simulink model "hcu_main_ADASwEPS"  (Simulink 8.2)
settings: Solver=FixedStepDiscrete  StartTime=0.0  StopTime=inf  FixedStep=0.001  RelTol=1e-3
PostLoadFcn:
  | , if any(exist('dsrtsu_mdlpostloadfcn', 'file') == [2, 3, 6]), try dsrtsu_mdlpostloadfcn('Execute', bdroot); catch fprintf('Error in PostLoadFcn (dsrtsu_mdlpostloadfcn) for model "%s":\n %s\n', bdroot, lasterr); end, end,
values from neighbouring files (symbols this model uses):
  C_TASK_1MS_S = (	C_TICK_TIME_S       )    [hcu_local_hdr.m]    (also in temp_ovrd_values.m = double(	0.001                  ))
  C_TICK_TIME_S = single(	0.005	    	)    [hcu_local_hdr.m]
  ENUM_EPSLFCSTATUS_ACTIVE = uint8(  2  )    [hcu_local_hdr.m]
  ENUM_EPSLFCSTATUS_TRANSITION = uint8(  3  )    [hcu_local_hdr.m]
  ENUM_EPSLKASTATUS_ACTIVE = uint8(  2  )    [hcu_local_hdr.m]
  ENUM_EPSMODEREQ_ANGLE = uint8(  1  )    [hcu_local_hdr.m]
  ENUM_EPSMODEREQ_INTERNAL = uint8(  0  )    [hcu_local_hdr.m]
  ENUM_EPSMODEREQ_TORQUE = uint8(  2  )    [hcu_local_hdr.m]
  ENUM_GEARPOSN_1ST = uint8(  1  )    [hcu_local_hdr.m]
  ENUM_GEARPOSN_2ND = uint8(  2  )    [hcu_local_hdr.m]
  ENUM_GEARPOSN_3RD = uint8(  3  )    [hcu_local_hdr.m]
  ENUM_GEARPOSN_4TH = uint8(  4  )    [hcu_local_hdr.m]
  ENUM_GEARPOSN_5TH = uint8(  5  )    [hcu_local_hdr.m]
  ENUM_GEARPOSN_6TH = uint8(  6  )    [hcu_local_hdr.m]
  ENUM_GEARPOSN_R = uint8(  7  )    [hcu_local_hdr.m]
  FALSE = boolean( 0 )    [hcu_local_hdr.m]
  TRUE = boolean( 1 )    [hcu_local_hdr.m]
undefined symbols (not defined in the file or in its folder): AISP_EPSCurrent_pct, AISP_TqASensorDelta_pct, AISP_TqBSensorDelta_pct, dHAL_IN, hal, INVALID_ABS1_TIMEOUT, INVALID_ABS2_TIMEOUT, INVALID_ABS3_TIMEOUT, INVALID_ABS4_TIMEOUT, INVALID_AC1_TIMEOUT, INVALID_ADASTORQ_REQ, INVALID_BCM1_TIMEOUT, INVALID_BCM2_TIMEOUT, INVALID_BOOSTER_VAC, INVALID_CSW1_TIMEOUT, INVALID_CUR_VEHDECE, INVALID_CURBRAKEDECE_REQ, INVALID_CURSTEERANG_REQ, INVALID_CURSTEERTQ_REQ, INVALID_ECM1_TIMEOUT, INVALID_ECM2_TIMEOUT, INVALID_ECM3_TIMEOUT, INVALID_ECM9_TIMEOUT, INVALID_ENG_TORQUE_FRICTIONAL, INVALID_ENG_TORQUE_INDICATED, INVALID_ENG_TORQUE_INDICATEDCOR, INVALID_ENG_TQ_MAX, INVALID_ENG_TQ_MIN, INVALID_EPAS2_TIMEOUT, INVALID_EPAS3_TIMEOUT, INVALID_EPB1_TIMEOUT, INVALID_EPS_BATTVOLT, INVALID_ESC_BATTVOLT, INVALID_GRADE, INVALID_HCU3_TIMEOUT, INVALID_HCU4_TIMEOUT, INVALID_HMI1_TIMEOUT, INVALID_HMI2_TIMEOUT, INVALID_LAT_ACC, INVALID_LONG_ACC, INVALID_MC_PRESSURE, INVALID_METER1_TIMEOUT, INVALID_METER3_TIMEOUT, INVALID_METER_VEHSPD, INVALID_ODO_METER, INVALID_OUTSIDE_TEMP, INVALID_PARKBRAKEBIND_STAT, INVALID_PEDALTQ_REQ, INVALID_SAS1_TIMEOUT, INVALID_SAS_ANGLE, INVALID_SHIFTER_POSN, INVALID_TCM1_TIMEOUT, INVALID_TCM2_TIMEOUT, INVALID_VCU1_TIMEOUT, INVALID_VCU2_TIMEOUT, INVALID_VEH_CRASH, INVALID_VEH_SPD, INVALID_WHEEL_SPD, INVALID_YAW_RATE, KHAL_MssgIdObj1_num ... (+8)
libraries: simulink x147, hcu_lib x38, rti1401lib_dio_type3 x4, rtimmsu_dsrtlib x3, app x1, rtiethernetudplib x1, rti1401lib_adc_type4 x1, rti1401lib_dac_type3 x1, inp x1, lidr x1, outp x1
(part 15 of 15)

== stateflow chart EPSS/EPSS/InternalMode/LKA_Flow_Chart ==
  state UNAVAILABLE
    VEPSS_EPSLKAStatus_enum=ENUM_EPSLKASTATUS_OFF;
  state AVAILABLE
    VEPSS_EPSLKAStatus_enum=ENUM_EPSLKASTATUS_READY;
  state PROGRESS
    VEPSS_EPSLKAStatus_enum=ENUM_EPSLKASTATUS_ACTIVE;
  state INVALID
    VEPSS_EPSLKAStatus_enum=ENUM_EPSLKASTATUS_NOTAVAIL_PERM;
  (default) -> UNAVAILABLE : {VEPSS_EPSLKAAbReason_enum= ...
      | ENUM_EPSADASABREASON_NO_DRIVING_INTERRUPTION;}
  AVAILABLE -> PROGRESS [order 2] : [VISP_ADASLKAStatus_enum==ENUM_ADASLKASTATUS_ACTIVE && ...
      | VISP_EPSModeReq_enum==ENUM_EPSMODEREQ_INTERNAL && ...
      | VISP_StrTqReqAppl_flg]
      | {VEPSS_EPSLKAAbReason_enum= ...
      | ENUM_EPSADASABREASON_NO_DRIVING_INTERRUPTION;}
  UNAVAILABLE -> AVAILABLE [order 1] : [VISP_ADASLKAStatus_enum==ENUM_ADASLKASTATUS_STANDBY && ...
      | VISP_EPSModeReq_enum==ENUM_EPSMODEREQ_INTERNAL]
      | {VEPSS_EPSLKAAbReason_enum= ...
      | ENUM_EPSADASABREASON_NO_DRIVING_INTERRUPTION;}
  PROGRESS -> AVAILABLE [order 1] : [VISP_EPSModeReq_enum==ENUM_EPSMODEREQ_INTERNAL && ...
      | (VISP_ADASLKAStatus_enum==ENUM_ADASLKASTATUS_STANDBY || ...
      | !VISP_StrTqReqAppl_flg)]
      | {VEPSS_EPSLKAAbReason_enum= ...
      | ENUM_EPSADASABREASON_NO_DRIVING_INTERRUPTION;}
  AVAILABLE -> UNAVAILABLE [order 1] : [(VISP_ADASLKAStatus_enum==ENUM_ADASLKASTATUS_OFF || ...
      | VISP_EPSModeReq_enum==ENUM_EPSMODEREQ_TORQUE || ...
      | VISP_EPSModeReq_enum==ENUM_EPSMODEREQ_ANGLE)]
      | {VEPSS_EPSLKAAbReason_enum= ...
      | ENUM_EPSADASABREASON_NO_DRIVING_INTERRUPTION;}
  (junction 314) -> UNAVAILABLE
  (junction 313) -> UNAVAILABLE
  UNAVAILABLE -> (junction 311) [order 2]
  AVAILABLE -> INVALID [order 3] : [VISP_ADASLKAStatus_enum==ENUM_ADASLKASTATUS_NOTAVAIL_TEMP || ...
      | VISP_ADASLKAStatus_enum==ENUM_ADASLKASTATUS_NOTAVAIL_PERM || ...
      | VISP_EPSModeReq_enum==ENUM_EPSMODEREQ_INVALID]
      | {VEPSS_EPSLKAAbReason_enum= ...
      | ENUM_EPSADASABREASON_OTHER_DEFAULT;}
  PROGRESS -> (junction 312) [order 2]
  PROGRESS -> (junction 315) [order 3]
  (junction 311) -> INVALID : [VISP_ADASLKAStatus_enum==ENUM_ADASLKASTATUS_NOTAVAIL_TEMP || ...
      | VISP_ADASLKAStatus_enum==ENUM_ADASLKASTATUS_NOTAVAIL_PERM || ...
      | VISP_EPSModeReq_enum==ENUM_EPSMODEREQ_INVALID]
      | {VEPSS_EPSLKAAbReason_enum= ...
      | ENUM_EPSADASABREASON_OTHER_DEFAULT;}
  (junction 312) -> INVALID : [VISP_ADASLKAStatus_enum==ENUM_ADASLKASTATUS_NOTAVAIL_TEMP || ...
      | VISP_ADASLKAStatus_enum==ENUM_ADASLKASTATUS_NOTAVAIL_PERM || ...
      | VISP_EPSModeReq_enum==ENUM_EPSMODEREQ_INVALID]
      | {VEPSS_EPSLKAAbReason_enum= ...
      | ENUM_EPSADASABREASON_OTHER_DEFAULT;}
  INVALID -> (junction 313) : [VISP_ADASLKAStatus_enum==ENUM_ADASLKASTATUS_OFF && ...
      | VEPSS_StrTqReqZERO_flg]
      | {VEPSS_EPSLKAAbReason_enum= ...
      | ENUM_EPSADASABREASON_NO_DRIVING_INTERRUPTION;}
  (junction 315) -> (junction 314) : [(VISP_ADASLKAStatus_enum==ENUM_ADASLKASTATUS_OFF || ...
      | VISP_EPSModeReq_enum==ENUM_EPSMODEREQ_TORQUE || ...
      | VISP_EPSModeReq_enum==ENUM_EPSMODEREQ_ANGLE)]
      | {VEPSS_EPSLKAAbReason_enum= ...
      | ENUM_EPSADASABREASON_NO_DRIVING_INTERRUPTION;}
  data: VEPSS_EPSLKAStatus_enum output uint8; ENUM_EPSLKASTATUS_OFF parameter double; ENUM_EPSLKASTATUS_READY parameter double; ENUM_EPSLKASTATUS_ACTIVE parameter double; ENUM_EPSLKASTATUS_NOTAVAIL_TEMP parameter double; ENUM_EPSLKASTATUS_NOTAVAIL_PERM parameter double; VISP_ADASLKAStatus_enum input double; ENUM_ADASLKASTATUS_OFF parameter double; ENUM_ADASLKASTATUS_STANDBY parameter double; ENUM_ADASLKASTATUS_ACTIVE parameter double; ENUM_ADASLKASTATUS_NOTAVAIL_TEMP parameter double; ENUM_ADASLKASTATUS_NOTAVAIL_PERM parameter double; VISP_EPSModeReq_enum input double; VEPSS_StrTqReqZERO_flg input double; ENUM_EPSMODEREQ_INTERNAL parameter double; ENUM_EPSMODEREQ_ANGLE parameter double; ENUM_EPSMODEREQ_TORQUE parameter double; ENUM_EPSMODEREQ_INVALID parameter double; VEPSS_EPSLKAAbReason_enum output uint8; ENUM_EPSADASABREASON_NO_DRIVING_INTERRUPTION parameter double; ENUM_EPSADASABREASON_THERMAL_ERROR parameter double; ENUM_EPSADASABREASON_GEAR_POSITION_ERROR parameter double; ENUM_EPSADASABREASON_VEHICLE_SPEED_ERROR parameter double; ENUM_EPSADASABREASON_DRIVER_RECOVERY parameter double; ENUM_EPSADASABREASON_TORQUE_ERROR parameter double; ENUM_EPSADASABREASON_REQUEST_TORQUE_ERROR parameter double; ENUM_EPSADASABREASON_THERMAL_PROTECTION parameter double; ENUM_EPSADASABREASON_TRANSITION_GAIN_ERROR parameter double; ENUM_EPSADASABREASON_OTHER_DEFAULT parameter double; VISP_StrTqReqAppl_flg input double

== stateflow chart EPSS/EPSS/TorqueMode/LFC_Flow_Chart ==
  state UNAVAILABLE
    VEPSS_EPSLFCStatus_enum=ENUM_EPSLFCSTATUS_OFF;
  state AVAILABLE
    VEPSS_EPSLFCStatus_enum=ENUM_EPSLFCSTATUS_READY;
  state PROGRESS_NORMAL
    VEPSS_EPSLFCStatus_enum=ENUM_EPSLFCSTATUS_ACTIVE;
  state INVALID
    VEPSS_EPSLFCStatus_enum=ENUM_EPSLFCSTATUS_NOTAVAIL_PERM;
  state PROGRESS_TRANSITION
    VEPSS_EPSLFCStatus_enum=ENUM_EPSLFCSTATUS_TRANSITION;
  (default) -> UNAVAILABLE : {VEPSS_EPSLFCAbReason_enum= ...
      | ENUM_EPSADASABREASON_NO_DRIVING_INTERRUPTION;}
  AVAILABLE -> PROGRESS_NORMAL [order 2] : [VISP_ADASLFCStatus_enum==ENUM_ADASLFCSTATUS_ACTIVE_NORMAL && ...
      | VISP_EPSModeReq_enum==ENUM_EPSMODEREQ_TORQUE && ...
      | VISP_StrTqReqAppl_flg]
      | {VEPSS_EPSLFCAbReason_enum= ...
      | ENUM_EPSADASABREASON_NO_DRIVING_INTERRUPTION;}
  UNAVAILABLE -> AVAILABLE [order 1] : [VISP_ADASLFCStatus_enum==ENUM_ADASLFCSTATUS_STANDBY]
      | {VEPSS_EPSLFCAbReason_enum= ...
      | ENUM_EPSADASABREASON_NO_DRIVING_INTERRUPTION;}
  PROGRESS_NORMAL -> (junction 371) [order 4] : [VISP_ADASLFCStatus_enum==ENUM_ADASLFCSTATUS_OFF]
      | {VEPSS_EPSLFCAbReason_enum= ...
      | ENUM_EPSADASABREASON_NO_DRIVING_INTERRUPTION;}
  (junction 371) -> (junction 386)
  PROGRESS_NORMAL -> AVAILABLE [order 1] : [(VISP_ADASLFCStatus_enum==ENUM_ADASLFCSTATUS_STANDBY || ...
      | VISP_EPSModeReq_enum==ENUM_EPSMODEREQ_INTERNAL || ...
      | VISP_EPSModeReq_enum==ENUM_EPSMODEREQ_ANGLE || ...
      | !VISP_StrTqReqAppl_flg)]
      | {VEPSS_EPSLFCAbReason_enum= ...
      | ENUM_EPSADASABREASON_NO_DRIVING_INTERRUPTION;}
  AVAILABLE -> UNAVAILABLE [order 1] : [VISP_ADASLFCStatus_enum==ENUM_ADASLFCSTATUS_OFF]
      | {VEPSS_EPSLFCAbReason_enum= ...
      | ENUM_EPSADASABREASON_NO_DRIVING_INTERRUPTION;}
  (junction 384) -> UNAVAILABLE
  (junction 382) -> UNAVAILABLE
  UNAVAILABLE -> (junction 378) [order 2]
  AVAILABLE -> (junction 374) [order 3]
  (junction 372) -> AVAILABLE
  PROGRESS_NORMAL -> (junction 379) [order 2]
  PROGRESS_NORMAL -> PROGRESS_TRANSITION [order 3] : [VISP_ADASLFCStatus_enum==ENUM_ADASLFCSTATUS_ACTIVE_TRANSITION && ...
      | VISP_EPSModeReq_enum==ENUM_EPSMODEREQ_TORQUE && ...
      | VISP_StrTqReqAppl_flg]
      | {VEPSS_EPSLFCAbReason_enum= ...
      | ENUM_EPSADASABREASON_NO_DRIVING_INTERRUPTION;}
  PROGRESS_TRANSITION -> (junction 372) [order 3] : [(VISP_ADASLFCStatus_enum==ENUM_ADASLFCSTATUS_STANDBY || ...
      | VISP_EPSModeReq_enum==ENUM_EPSMODEREQ_INTERNAL || ...
      | VISP_EPSModeReq_enum==ENUM_EPSMODEREQ_ANGLE || ...
      | !VISP_StrTqReqAppl_flg)]
      | {VEPSS_EPSLFCAbReason_enum= ...
      | ENUM_EPSADASABREASON_NO_DRIVING_INTERRUPTION;}
  PROGRESS_TRANSITION -> (junction 373) [order 1] : [VISP_ADASLFCStatus_enum==ENUM_ADASLFCSTATUS_OFF]
      | {VEPSS_EPSLFCAbReason_enum= ...
      | ENUM_EPSADASABREASON_NO_DRIVING_INTERRUPTION;}
  (junction 373) -> (junction 385)
  (junction 374) -> (junction 375) [order 1] : [!VEPSS_LFCTransGainONE_flg]
      | {VEPSS_EPSLFCAbReason_enum= ...
      | ENUM_EPSADASABREASON_TRANSITION_GAIN_ERROR;}
  (junction 374) -> (junction 376) [order 2]
  (junction 375) -> (junction 377)
  PROGRESS_TRANSITION -> (junction 383) [order 2]
  (junction 376) -> (junction 377) : [VISP_ADASLFCStatus_enum==ENUM_ADASLFCSTATUS_NOTAVAIL_TEMP || ...
      | VISP_ADASLFCStatus_enum==ENUM_ADASLFCSTATUS_NOTAVAIL_PERM || ...
      | VISP_EPSModeReq_enum==ENUM_EPSMODEREQ_INVALID]
      | {VEPSS_EPSLFCAbReason_enum= ...
      | ENUM_EPSADASABREASON_OTHER_DEFAULT;}
  (junction 377) -> INVALID
  (junction 378) -> INVALID [order 1] : [!VEPSS_LFCTransGainONE_flg]
      | {VEPSS_EPSLFCAbReason_enum= ...
      | ENUM_EPSADASABREASON_TRANSITION_GAIN_ERROR;}
  (junction 379) -> INVALID [order 1] : [!VEPSS_LFCTransGainONE_flg]
      | {VEPSS_EPSLFCAbReason_enum= ...
      | ENUM_EPSADASABREASON_TRANSITION_GAIN_ERROR;}
  (junction 378) -> (junction 380) [order 2]
  (junction 379) -> (junction 381) [order 2]
  (junction 380) -> INVALID : [VISP_ADASLFCStatus_enum==ENUM_ADASLFCSTATUS_NOTAVAIL_TEMP || ...
      | VISP_ADASLFCStatus_enum==ENUM_ADASLFCSTATUS_NOTAVAIL_PERM || ...
      | VISP_EPSModeReq_enum==ENUM_EPSMODEREQ_INVALID]
      | {VEPSS_EPSLFCAbReason_enum= ...
      | ENUM_EPSADASABREASON_OTHER_DEFAULT;}
  (junction 381) -> INVALID : [VISP_ADASLFCStatus_enum==ENUM_ADASLFCSTATUS_NOTAVAIL_TEMP || ...
      | VISP_ADASLFCStatus_enum==ENUM_ADASLFCSTATUS_NOTAVAIL_PERM || ...
      | VISP_EPSModeReq_enum==ENUM_EPSMODEREQ_INVALID]
      | {VEPSS_EPSLFCAbReason_enum= ...
      | ENUM_EPSADASABREASON_OTHER_DEFAULT;}
  INVALID -> (junction 382) : [VISP_ADASLFCStatus_enum==ENUM_ADASLFCSTATUS_OFF && ...
      | VEPSS_StrTqReqZERO_flg && ...
      | VEPSS_LFCTransGainONE_flg]
      | {VEPSS_EPSLFCAbReason_enum= ...
      | ENUM_EPSADASABREASON_NO_DRIVING_INTERRUPTION;}
  (junction 383) -> INVALID : [VISP_ADASLFCStatus_enum==ENUM_ADASLFCSTATUS_NOTAVAIL_TEMP || ...
      | VISP_ADASLFCStatus_enum==ENUM_ADASLFCSTATUS_NOTAVAIL_PERM || ...
      | VISP_EPSModeReq_enum==ENUM_EPSMODEREQ_INVALID]
      | {VEPSS_EPSLFCAbReason_enum= ...
      | ENUM_EPSADASABREASON_OTHER_DEFAULT;}
  (junction 385) -> (junction 384)
  (junction 386) -> (junction 385)
  data: VEPSS_EPSLFCStatus_enum output uint8; ENUM_EPSLFCSTATUS_OFF parameter double; ENUM_EPSLFCSTATUS_READY parameter double; ENUM_EPSLFCSTATUS_ACTIVE parameter double; ENUM_EPSLFCSTATUS_NOTAVAIL_TEMP parameter double; ENUM_EPSLFCSTATUS_NOTAVAIL_PERM parameter double; VISP_ADASLFCStatus_enum input double; ENUM_ADASLFCSTATUS_OFF parameter double; ENUM_ADASLFCSTATUS_STANDBY parameter double; ENUM_ADASLFCSTATUS_ACTIVE_NORMAL parameter double; ENUM_ADASLFCSTATUS_NOTAVAIL_TEMP parameter double; ENUM_ADASLFCSTATUS_NOTAVAIL_PERM parameter double; VISP_EPSModeReq_enum input double; VISP_StrTqReqAppl_flg input double; VEPSS_StrTqReqZERO_flg input double; ENUM_EPSMODEREQ_INTERNAL parameter double; ENUM_EPSMODEREQ_ANGLE parameter double; ENUM_EPSMODEREQ_TORQUE parameter double; ENUM_EPSMODEREQ_INVALID parameter double; VEPSS_EPSLFCAbReason_enum output uint8; ENUM_EPSADASABREASON_NO_DRIVING_INTERRUPTION parameter double; ENUM_EPSADASABREASON_THERMAL_ERROR parameter double; ENUM_EPSADASABREASON_GEAR_POSITION_ERROR parameter double; ENUM_EPSADASABREASON_VEHICLE_SPEED_ERROR parameter double; ENUM_EPSADASABREASON_DRIVER_RECOVERY parameter double; ENUM_EPSADASABREASON_TORQUE_ERROR parameter double; ENUM_EPSADASABREASON_REQUEST_TORQUE_ERROR parameter double; ENUM_EPSADASABREASON_THERMAL_PROTECTION parameter double; ENUM_EPSADASABREASON_TRANSITION_GAIN_ERROR parameter double; ENUM_EPSADASABREASON_OTHER_DEFAULT parameter double; ENUM_EPSLFCSTATUS_TRANSITION parameter double; ENUM_ADASLFCSTATUS_ACTIVE_TRANSITION parameter double; VEPSS_LFCTransGainONE_flg input double

== stateflow chart EPSS/EPSS/AngleMode/LFC_Flow_Chart ==
  state UNAVAILABLE
    VEPSS_EPSLFCStatus_enum=ENUM_EPSLFCSTATUS_OFF;
  state AVAILABLE
    VEPSS_EPSLFCStatus_enum=ENUM_EPSLFCSTATUS_READY;
  state PROGRESS_NORMAL
    VEPSS_EPSLFCStatus_enum=ENUM_EPSLFCSTATUS_ACTIVE;
  state INVALID
    VEPSS_EPSLFCStatus_enum=ENUM_EPSLFCSTATUS_NOTAVAIL_PERM;
  state PROGRESS_TRANSITION
    VEPSS_EPSLFCStatus_enum=ENUM_EPSLFCSTATUS_TRANSITION;
  (default) -> UNAVAILABLE : {VEPSS_EPSLFCAbReason_enum= ...
      | ENUM_EPSADASABREASON_NO_DRIVING_INTERRUPTION;}
  AVAILABLE -> PROGRESS_NORMAL [order 2] : [VISP_ADASLFCStatus_enum==ENUM_ADASLFCSTATUS_ACTIVE_NORMAL && ...
      | VISP_EPSModeReq_enum==ENUM_EPSMODEREQ_ANGLE && ...
      | VISP_StrAngReqAppl_flg]
      | {VEPSS_EPSLFCAbReason_enum= ...
      | ENUM_EPSADASABREASON_NO_DRIVING_INTERRUPTION;}
  UNAVAILABLE -> AVAILABLE [order 1] : [VISP_ADASLFCStatus_enum==ENUM_ADASLFCSTATUS_STANDBY]
      | {VEPSS_EPSLFCAbReason_enum= ...
      | ENUM_EPSADASABREASON_NO_DRIVING_INTERRUPTION;}
  PROGRESS_NORMAL -> (junction 459) [order 4] : [VISP_ADASLFCStatus_enum==ENUM_ADASLFCSTATUS_OFF]
      | {VEPSS_EPSLFCAbReason_enum= ...
      | ENUM_EPSADASABREASON_NO_DRIVING_INTERRUPTION;}
  (junction 459) -> (junction 470)
  PROGRESS_NORMAL -> AVAILABLE [order 1] : [(VISP_ADASLFCStatus_enum==ENUM_ADASLFCSTATUS_STANDBY || ...
      | VISP_EPSModeReq_enum==ENUM_EPSMODEREQ_INTERNAL || ...
      | VISP_EPSModeReq_enum==ENUM_EPSMODEREQ_TORQUE || ...
      | !VISP_StrAngReqAppl_flg)]
      | {VEPSS_EPSLFCAbReason_enum= ...
      | ENUM_EPSADASABREASON_NO_DRIVING_INTERRUPTION;}
  AVAILABLE -> UNAVAILABLE [order 1] : [VISP_ADASLFCStatus_enum==ENUM_ADASLFCSTATUS_OFF]
      | {VEPSS_EPSLFCAbReason_enum= ...
      | ENUM_EPSADASABREASON_NO_DRIVING_INTERRUPTION;}
  (junction 468) -> UNAVAILABLE
  (junction 466) -> UNAVAILABLE
  UNAVAILABLE -> (junction 464) [order 2]
  AVAILABLE -> (junction 462) [order 3]
  (junction 460) -> AVAILABLE
  PROGRESS_NORMAL -> (junction 465) [order 3]
  PROGRESS_NORMAL -> PROGRESS_TRANSITION [order 2] : [VISP_ADASLFCStatus_enum==ENUM_ADASLFCSTATUS_ACTIVE_TRANSITION && ...
      | VISP_EPSModeReq_enum==ENUM_EPSMODEREQ_ANGLE && ...
      | VISP_StrAngReqAppl_flg]
      | {VEPSS_EPSLFCAbReason_enum= ...
      | ENUM_EPSADASABREASON_NO_DRIVING_INTERRUPTION;}
  PROGRESS_TRANSITION -> (junction 460) [order 3] : [(VISP_ADASLFCStatus_enum==ENUM_ADASLFCSTATUS_STANDBY || ...
      | VISP_EPSModeReq_enum==ENUM_EPSMODEREQ_INTERNAL || ...
      | VISP_EPSModeReq_enum==ENUM_EPSMODEREQ_TORQUE || ...
      | !VISP_StrAngReqAppl_flg)]
      | {VEPSS_EPSLFCAbReason_enum= ...
      | ENUM_EPSADASABREASON_NO_DRIVING_INTERRUPTION;}
  PROGRESS_TRANSITION -> (junction 461) [order 1] : [VISP_ADASLFCStatus_enum==ENUM_ADASLFCSTATUS_OFF]
      | {VEPSS_EPSLFCAbReason_enum= ...
      | ENUM_EPSADASABREASON_NO_DRIVING_INTERRUPTION;}
  (junction 461) -> (junction 469)
  PROGRESS_TRANSITION -> (junction 467) [order 2]
  (junction 462) -> (junction 463) : [VISP_ADASLFCStatus_enum==ENUM_ADASLFCSTATUS_NOTAVAIL_TEMP || ...
      | VISP_ADASLFCStatus_enum==ENUM_ADASLFCSTATUS_NOTAVAIL_PERM || ...
      | VISP_EPSModeReq_enum==ENUM_EPSMODEREQ_INVALID]
      | {VEPSS_EPSLFCAbReason_enum= ...
      | ENUM_EPSADASABREASON_OTHER_DEFAULT;}
  (junction 463) -> INVALID
  (junction 464) -> INVALID : [VISP_ADASLFCStatus_enum==ENUM_ADASLFCSTATUS_NOTAVAIL_TEMP || ...
      | VISP_ADASLFCStatus_enum==ENUM_ADASLFCSTATUS_NOTAVAIL_PERM || ...
      | VISP_EPSModeReq_enum==ENUM_EPSMODEREQ_INVALID]
      | {VEPSS_EPSLFCAbReason_enum= ...
      | ENUM_EPSADASABREASON_OTHER_DEFAULT;}
  (junction 465) -> INVALID : [VISP_ADASLFCStatus_enum==ENUM_ADASLFCSTATUS_NOTAVAIL_TEMP || ...
      | VISP_ADASLFCStatus_enum==ENUM_ADASLFCSTATUS_NOTAVAIL_PERM || ...
      | VISP_EPSModeReq_enum==ENUM_EPSMODEREQ_INVALID]
      | {VEPSS_EPSLFCAbReason_enum= ...
      | ENUM_EPSADASABREASON_OTHER_DEFAULT;}
  INVALID -> (junction 466) : [VISP_ADASLFCStatus_enum==ENUM_ADASLFCSTATUS_OFF && ...
      | VEPSS_StrAngReqZERO_flg]
      | {VEPSS_EPSLFCAbReason_enum= ...
      | ENUM_EPSADASABREASON_NO_DRIVING_INTERRUPTION;}
  (junction 467) -> INVALID : [VISP_ADASLFCStatus_enum==ENUM_ADASLFCSTATUS_NOTAVAIL_TEMP || ...
      | VISP_ADASLFCStatus_enum==ENUM_ADASLFCSTATUS_NOTAVAIL_PERM || ...
      | VISP_EPSModeReq_enum==ENUM_EPSMODEREQ_INVALID]
      | {VEPSS_EPSLFCAbReason_enum= ...
      | ENUM_EPSADASABREASON_OTHER_DEFAULT;}
  (junction 469) -> (junction 468)
  (junction 470) -> (junction 469)
  data: VEPSS_EPSLFCStatus_enum output uint8; ENUM_EPSLFCSTATUS_OFF parameter double; ENUM_EPSLFCSTATUS_READY parameter double; ENUM_EPSLFCSTATUS_ACTIVE parameter double; ENUM_EPSLFCSTATUS_NOTAVAIL_TEMP parameter double; ENUM_EPSLFCSTATUS_NOTAVAIL_PERM parameter double; VISP_ADASLFCStatus_enum input double; ENUM_ADASLFCSTATUS_OFF parameter double; ENUM_ADASLFCSTATUS_STANDBY parameter double; ENUM_ADASLFCSTATUS_ACTIVE_NORMAL parameter double; ENUM_ADASLFCSTATUS_NOTAVAIL_TEMP parameter double; ENUM_ADASLFCSTATUS_NOTAVAIL_PERM parameter double; VISP_EPSModeReq_enum input double; VISP_StrAngReqAppl_flg input double; VEPSS_StrAngReqZERO_flg input double; ENUM_EPSMODEREQ_INTERNAL parameter double; ENUM_EPSMODEREQ_ANGLE parameter double; ENUM_EPSMODEREQ_TORQUE parameter double; ENUM_EPSMODEREQ_INVALID parameter double; VEPSS_EPSLFCAbReason_enum output uint8; ENUM_EPSADASABREASON_NO_DRIVING_INTERRUPTION parameter double; ENUM_EPSADASABREASON_THERMAL_ERROR parameter double; ENUM_EPSADASABREASON_GEAR_POSITION_ERROR parameter double; ENUM_EPSADASABREASON_VEHICLE_SPEED_ERROR parameter double; ENUM_EPSADASABREASON_DRIVER_RECOVERY parameter double; ENUM_EPSADASABREASON_TORQUE_ERROR parameter double; ENUM_EPSADASABREASON_REQUEST_TORQUE_ERROR parameter double; ENUM_EPSADASABREASON_THERMAL_PROTECTION parameter double; ENUM_EPSADASABREASON_TRANSITION_GAIN_ERROR parameter double; ENUM_EPSADASABREASON_OTHER_DEFAULT parameter double; ENUM_EPSLFCSTATUS_TRANSITION parameter double; ENUM_ADASLFCSTATUS_ACTIVE_TRANSITION parameter double
